simulink library "ddm"  (R2021b)
settings: Solver=VariableStepAuto  StartTime=0.0  StopTime=10.0  RelTol=1e-3
undefined symbols (not defined in the file or in its folder): ENUM_ADASACCSTA_ERROR, ENUM_ADASACCSTA_OFF, ENUM_ADASACCSTA_STANDBY, ENUM_ADASISASTA_OFF, ENUM_ALLOWMOV_ALLOWREADY, ENUM_APS, ENUM_BRKSTA_ERROR, ENUM_BRKSTA_OFF, ENUM_BRKSTA_ON, ENUM_CHGPREACTERRSTA_OBCPRE, ENUM_DCDCFAULTSTA_ANYFAULTLV1, ENUM_DCDCFAULTSTA_ANYFAULTLV2, ENUM_DRIVETRAIN_AWD, ENUM_DRIVETRAIN_FWD, ENUM_DRIVETRAIN_RWD, ENUM_DRSEATSTA_INVALID, ENUM_EDUDRTSTA_NORMAL, ENUM_EPBSTA_APPLIED, ENUM_EPBSTA_RELEASED, ENUM_HVBATTREADYPRE_READY, ENUM_MCUWARN_LV0, ENUM_MCUWARN_LV1, ENUM_MCUWARN_LV2, ENUM_MCUWARN_LV3, ENUM_MCUWARN_NOERROR, ENUM_OBCFAULTSTA_ANYFAULT, ENUM_PAS_R2F2, ENUM_PDFAULT_BATTPDFAIL, ENUM_PDFAULT_DCDCDISABLE, ENUM_PDFAULT_MCUDISABLE, ENUM_PDFAULT_MCUDISCHRG, ENUM_POWERSTA_OFF, ENUM_POWERSTA_ON, ENUM_POWERSTA_READY, ENUM_POWERSTA_STANDBY, ENUM_PRESSINDI_LOW, ENUM_PUFAULT_BATTUPFAIL, ENUM_PUFAULT_DCDCENABLEFAIL, ENUM_PUFAULT_PRECHRGCHKFAIL, ENUM_PUFAULT_SAFETYCHKFAIL, ENUM_PUSTATE_COMPLETED, ENUM_PWRSTASW_OFF, ENUM_PWRSTASW_OFFA, ENUM_PWRSTASW_OFFCHVCHRG, ENUM_PWRSTASW_OFFCLVCHRG, ENUM_PWRSTASW_ON, ENUM_PWRSTASW_ONHVCHRG, ENUM_PWRSTASW_READY, ENUM_PWRSTASW_STANDBY, ENUM_RANGESTA_12IN, ENUM_RANGESTA_12OUT, ENUM_SHIFTCOMMAND_D, ENUM_SHIFTCOMMAND_N, ENUM_SHIFTCOMMAND_P, ENUM_SHIFTCOMMAND_R, ENUM_ZONEMALFUNLV_1ST, ENUM_ZONEMALFUNLV_2ND, ENUM_ZONEMALFUNLV_3RD, ENUM_ZONEMALFUNLV_4TH, ENUM_ZONESPDCTRLMODE_ACC ... (+832)
libraries: hcu_lib x738, $bdroot x26, simulink x7
(part 17 of 25)

== system ddm/DDM/DDM/PMM/SW failure/FR Door switch failure ==
  note: Fail Safe During Detection
  note: Fail Safe After Decision
  note: Release Condition After Decision
  note: Release Condition During Detection
  note: Diagnostics and Fault Handling
  note: Test Detection Criteria
  note: Test Pass Criteria
  task_time_s : Inport
  VPMM_PowerSta_enum : Inport  Port=2
  VPMM_PwrStaSW_enum : Inport  Port=3
  VINP_FRAJARSW : Inport  Port=4
  DTC_clear_request : Inport  Port=5
  Add2 : Sum
  Add3 : Sum
  Add4 : Sum  AccumDataTypeStr=uint16
  Constant{1..2,12..13,31} (5 alike) : Constant  Value=ZERO_INT
  Constant14 : Constant  Value=KDDM_FRDoorSW_s
  Constant28 : Constant  Value=ZERO_FLOAT
  Constant29 : Constant  Value=ONE_INT
  Constant3 : Constant  Value=ONE_INT
  Constant37 : Constant  Value=ENUM_PWRSTASW_OFF
  Constant39 : Constant  Value=KDDM_FRDoorSWPassTO_s
  Constant4 : Constant  Value=KDDM_FRDoorSW_s
  Constant{42,47,52,54} (4 alike) : Constant  Value=TRUE
  Constant45 : Constant  Value=ENUM_POWERSTA_OFF
  Constant49 : Constant  Value=KDDM_FRDoorSW_s
  Constant5 : Constant  Value=KDDM_FRDoorSWDTC_cnt
  Constant50 : Constant  Value=ENUM_PWRSTASW_OFF
  Constant53 : Constant  Value=FALSE
  Constant55 : Constant  Value=FALSE
  Constant56 : Constant  Value=KDDM_FRDoorSWPassSW_flg
  Constant57 : Constant  Value=KDDM_FRDoorSWCFSSW_flg
  Constant58 : Constant  Value=KDDM_FRDoorSWDFSSW_flg
  Constant59 : Constant  Value=KDDM_FRDoorSWDetSW_flg
  Constant6 : Constant  Value=KDDM_FRDoorSWDetTO_s
  Constant60 : Constant  Value=KDDM_FRDoorSWDTC_cnt
  Constant7 : Constant  Value=KDDM_FRDoorSWPassTO_s
  Constant8 : Constant  Value=KDDM_FRDoorSWDetTO_s
  Constant9 : Constant  Value=FALSE
  DTC_Couter1 : hcu_lib/Basic_Blocks/DTC_Couter
  DTC_Info : hcu_lib/Basic_Blocks/DTC_Info
  Data Type Conversion : DataTypeConversion  OutDataTypeStr=uint8
  Data Type Conversion{1..2,7..9} (5 alike) : DataTypeConversion
  Data Type Conversion3 : DataTypeConversion  OutDataTypeStr=uint16
  Data Type Conversion4 : DataTypeConversion  OutDataTypeStr=uint8
  Data Type Conversion5 : DataTypeConversion  OutDataTypeStr=uint32
  Data Type Conversion6 : DataTypeConversion  OutDataTypeStr=uint16
  Divide{,1,7,11,16,20} (6 alike) : Product  Inputs=*/
  Equal10 : RelationalOperator  Operator=~=  OutDataTypeStr=boolean  RndMeth=Simplest
  Equal13 : RelationalOperator  Operator=~=  OutDataTypeStr=boolean  RndMeth=Simplest
  Equal8 : RelationalOperator  Operator===  OutDataTypeStr=boolean  RndMeth=Simplest
  Equal9 : RelationalOperator  Operator=~=  OutDataTypeStr=boolean  RndMeth=Simplest
  Logical Operator1 : Logic  Operator=NOT  AllPortsSameDT=off  OutDataTypeStr=boolean
  Logical Operator{25,28..31} (5 alike) : Logic  AllPortsSameDT=off  OutDataTypeStr=boolean
  Logical Operator27 : Logic  Operator=OR  AllPortsSameDT=off  OutDataTypeStr=boolean
  Logical Operator32 : Logic  Operator=OR  AllPortsSameDT=off  OutDataTypeStr=boolean
  Logical Operator33 : Logic  Operator=OR  AllPortsSameDT=off  OutDataTypeStr=boolean
  Relational Operator : RelationalOperator  Operator=>  OutDataTypeStr=boolean  RndMeth=Simplest
  Relational Operator1 : RelationalOperator  Operator=<=  OutDataTypeStr=boolean  RndMeth=Simplest
  Relational Operator12 : RelationalOperator  OutDataTypeStr=boolean  RndMeth=Simplest
  Relational Operator13 : RelationalOperator  Operator=<  OutDataTypeStr=boolean  RndMeth=Simplest
  Relational Operator2 : RelationalOperator  Operator=>  OutDataTypeStr=boolean  RndMeth=Simplest
  Relational Operator8 : RelationalOperator  Operator=<  OutDataTypeStr=boolean  RndMeth=Simplest
  Relational Operator9 : RelationalOperator  Operator=<=  OutDataTypeStr=boolean  RndMeth=Simplest
  Relay1 : Relay  OnSwitchValue=ONE_INT  OffSwitchValue=ZERO_INT
  SR_Latch2 : hcu_lib/Basic_Blocks/SR_Latch
  SR_Latch5 : hcu_lib/Basic_Blocks/SR_Latch
  Switch{1..3,6,8..9,13} (7 alike) : Switch  Criteria=u2 > Threshold
  Switch{4,7,11..12,15..16} (6 alike) : Switch  Criteria=u2 ~= 0
  Test Detection Criteria1 : hcu_lib/Basic_Blocks/Test Detection Criteria
  Unit Delay{1..3,5..6} (5 alike) : UnitDelay  SampleTime=-1  HasFrameUpgradeWarning=on
  VDDM_FRDoorSWDTC_raw32 : Outport
  VCUFRDoorSta : Outport  Port=2
  wires:
  DTC_clear_request/1 -> [DTC_clear_request]
  VINP_FRAJARSW/1 -> [VINP_FR_AJAR_SW]
  task_time_s/1 -> [task_time_s]
  [VDDM_FRDoorSWCFS_flg] -> Switch11/2
  Constant42/1 -> Switch11/1
  Switch11/1 -> [VCUFRDoorSta]
  Logical Operator27/1 -> Switch15/2
  Constant52/1 -> Switch16/1
  Equal8/1 -> Logical Operator27/1
  [VDDM_FRDoorSWPass_flg] -> Switch16/2
  Constant53/1 -> Switch16/3
  Constant45/1 -> Equal8/2
  Constant55/1 -> Switch15/3
  Switch15/1 -> [VDDM_FRDoorSWCFSRls_flg]
  Switch16/1 -> [VDDM_FRDoorSWDFSRls_flg]
  [DTC_clear_request] -> Logical Operator27/2
  Constant54/1 -> Switch15/1
  [VPMM_PowerSta_enum] -> Equal8/1
  Relay1/1 -> SR_Latch2/1
  [VDDM_FRDoorSWDet_flg] -> Logical Operator31/1
  Logical Operator29/1 -> DTC_Couter1/2
  [VDDM_FRDoorSWCFSRls_flg] -> SR_Latch5/2
  SR_Latch2/1 -> Logical Operator28/2
  SR_Latch5/1 -> Logical Operator30/1
  [VDDM_FRDoorSWDFSRls_flg] -> Logical Operator32/1
  Logical Operator32/1 -> SR_Latch2/2
  DTC_Couter1/2 -> Data Type Conversion4/1
  Logical Operator33/1 -> Logical Operator29/1
  Data Type Conversion4/1 -> [VDDM_FRDoorSWDTC_cnt]  "VDDM_FRDoorSWDTC_cnt"
  [VDDM_FRDoorSWDTC_cnt] -> Relay1/1
  Logical Operator31/1 -> DTC_Couter1/1
  [VDDM_FRDoorSWCFS_flg] -> Logical Operator32/2
  Constant57/1 -> Logical Operator30/2
  DTC_Couter1/1 -> SR_Latch5/1
  Constant59/1 -> Logical Operator31/2
  [VDDM_FRDoorSWCFSRls_flg] -> Logical Operator33/2
  Logical Operator28/1 -> [VDDM_FRDoorSWDFS_flg]
  [VDDM_FRDoorSWPass_flg] -> Logical Operator33/1
  Logical Operator30/1 -> [VDDM_FRDoorSWCFS_flg]
  Constant56/1 -> Logical Operator29/2
  Constant60/1 -> DTC_Couter1/3
  Constant58/1 -> Logical Operator28/1
  [VCUFRDoorSta] -> VCUFRDoorSta/1
  Divide1/1 -> Relational Operator1/2
  Data Type Conversion5/1 -> [VDDM_FRDoorSWHiLoCount_enum]
  Relational Operator1/1 -> [VDDM_FRDoorSWFailcntEN_flg]
  Divide20/1 -> Data Type Conversion9/1
  Add2/1 -> Switch6/3
  [VINP_FR_AJAR_SW] -> Relational Operator/1
  Relational Operator2/1 -> Switch1/2
  Constant31/1 -> Switch6/1
  Unit Delay3/1 -> Equal10/1
  Equal10/1 -> [VDDM_FRDoorSWChange_flg]
  Constant1/1 -> Switch7/3
  Constant29/1 -> Add2/2
  Switch6/1 -> Unit Delay1/1
  Unit Delay1/1 -> Data Type Conversion5/1
  Constant12/1 -> Switch1/1
  Constant37/1 -> Equal13/2
  Switch2/1 -> Data Type Conversion2/1
  Add3/1 -> Data Type Conversion8/1
  Constant4/1 -> Divide/1
  Switch9/1 -> Switch8/1
  Equal13/1 -> Switch7/2
  [VDDM_FRDoorSWfail_cnt] -> Switch1/3
  [VPMM_PwrStaSW_enum] -> Equal13/1
  Switch7/1 -> Unit Delay5/1
  [VDDM_FRDoorSWHiLoCount_enum] -> Relational Operator2/1
  [VDDM_FRDoorSWFailcntEN_flg] -> Switch9/2
  Switch1/1 -> Switch8/3
  Test Detection Criteria1/1 -> [VDDM_FRDoorSWDet_flg]  "VDDM_FRDoorSWDet_flg"
  [VDDM_FRDoorSWHiLoCount_enum] -> Add3/1
  [VDDM_FRDoorSWChange_flg] -> Switch6/2
  [VDDM_FRDoorSWfail_cnt] -> Switch2/1, Relational Operator8/1
  Constant13/1 -> Switch9/3
  Constant14/1 -> Divide1/1
  Relational Operator/1 -> Unit Delay3/1, Equal10/2
  Constant28/1 -> Relational Operator/2
  Constant6/1 -> Divide20/1
  [VDDM_FRDoorSWChange_flg] -> Switch8/2
  Switch8/1 -> Switch7/1
  Divide/1 -> Relational Operator2/2
  Unit Delay5/1 -> Switch4/3, Data Type Conversion7/1
  Unit Delay2/1 -> Relational Operator9/1
  Switch12/1 -> Unit Delay6/1
  Constant3/1 -> Add4/1
  Relational Operator9/1 -> Logical Operator25/2
  Data Type Conversion6/1 -> Relational Operator12/1, [VDDM_FRDoorSWPass_cnt]
  [VDDM_FRDoorSWChange_flg] -> Logical Operator25/1
  Switch3/1 -> Data Type Conversion3/1
  Constant2/1 -> Switch13/3
  [VDDM_FRDoorSWPass_cnt] -> Switch3/1, Relational Operator13/1
  Divide11/1 -> Relational Operator12/2
  Logical Operator1/1 -> Switch13/2
  Logical Operator25/1 -> Logical Operator1/1
  Data Type Conversion/1 -> Switch12/3
  Divide16/1 -> Data Type Conversion1/1
  Constant7/1 -> Divide11/1
  Data Type Conversion3/1 -> Add4/2
  Add4/1 -> Switch13/1
  Equal9/1 -> Switch12/2
  Relational Operator12/1 -> [VDDM_FRDoorSWPass_flg]
  Switch13/1 -> Switch12/1
  Divide7/1 -> Relational Operator9/2
  [VPMM_PwrStaSW_enum] -> Equal9/1
  Constant50/1 -> Equal9/2
  Unit Delay6/1 -> Data Type Conversion6/1
  Constant47/1 -> Data Type Conversion/1
  Constant49/1 -> Divide7/1
  Constant39/1 -> Divide16/1
  [VDDM_FRDoorSWHiLoCount_enum] -> Unit Delay2/1
  VPMM_PowerSta_enum/1 -> [VPMM_PowerSta_enum]
  VPMM_PwrStaSW_enum/1 -> [VPMM_PwrStaSW_enum]
  [VINP_FR_AJAR_SW] -> Switch11/3
  Data Type Conversion9/1 -> Switch2/3, Relational Operator8/2
  Relational Operator8/1 -> Switch2/2
  Data Type Conversion2/1 -> Add3/2
  [VDDM_FRDoorSWHiLoCount_enum] -> Add2/1
  [VDDM_FRDoorSWHiLoCount_enum] -> Relational Operator1/1
  Data Type Conversion7/1 -> [VDDM_FRDoorSWfail_cnt]
  Relational Operator13/1 -> Switch3/2
  Data Type Conversion1/1 -> Switch3/3, Relational Operator13/2
  Data Type Conversion8/1 -> Switch9/1
  DTC_Info/1 -> VDDM_FRDoorSWDTC_raw32/1  "VDDM_FRDoorSWDTC_raw32"
  [VDDM_FRDoorSWPass_flg] -> DTC_Info/2
  [VDDM_FRDoorSWCFS_flg] -> DTC_Info/3
  [VDDM_FRDoorSWDet_flg] -> DTC_Info/1
  [task_time_s] -> Divide1/2
  [task_time_s] -> Divide20/2
  [task_time_s] -> Divide/2
  [task_time_s] -> Divide16/2
  [task_time_s] -> Divide7/2
  [task_time_s] -> Divide11/2
  [task_time_s] -> Test Detection Criteria1/2
  Constant8/1 -> Test Detection Criteria1/4
  Constant5/1 -> Test Detection Criteria1/3
  [DTC_clear_request] -> DTC_Info/4
  [DTC_clear_request] -> Switch4/2
  Switch4/1 -> Test Detection Criteria1/1
  Constant9/1 -> Switch4/1

== system ddm/DDM/DDM/PMM/SW failure/Hood switch failure ==
  note: Test Pass Criteria
  note: Test Detection Criteria
  note: Diagnostics and Fault Handling
  note: Release Condition During Detection
  note: Release Condition After Decision
  note: Fail Safe After Decision
  note: Fail Safe During Detection
  task_time_s : Inport
  VPMM_PowerSta_enum : Inport  Port=2
  VPMM_PwrStaSW_enum : Inport  Port=3
  VINP_HoodSW : Inport  Port=4
  DTC_clear_request : Inport  Port=5
  Add2 : Sum
  Add3 : Sum
  Add4 : Sum  AccumDataTypeStr=uint16
  Constant{1..2,12..13,31} (5 alike) : Constant  Value=ZERO_INT
  Constant14 : Constant  Value=KDDM_HoodSW_s
  Constant28 : Constant  Value=ZERO_FLOAT
  Constant29 : Constant  Value=ONE_INT
  Constant3 : Constant  Value=ONE_INT
  Constant37 : Constant  Value=ENUM_PWRSTASW_OFF
  Constant39 : Constant  Value=KDDM_HoodSWPassTO_s
  Constant4 : Constant  Value=KDDM_HoodSW_s
  Constant{42,47,52,54} (4 alike) : Constant  Value=TRUE
  Constant45 : Constant  Value=ENUM_POWERSTA_OFF
  Constant49 : Constant  Value=KDDM_HoodSW_s
  Constant5 : Constant  Value=KDDM_HoodSWPassTO_s
  Constant50 : Constant  Value=ENUM_PWRSTASW_OFF
  Constant53 : Constant  Value=FALSE
  Constant55 : Constant  Value=FALSE
  Constant56 : Constant  Value=KDDM_HoodSWPassSW_flg
  Constant57 : Constant  Value=KDDM_HoodSWCFSSW_flg
  Constant58 : Constant  Value=KDDM_HoodSWDFSSW_flg
  Constant59 : Constant  Value=KDDM_HoodSWDetSW_flg
  Constant6 : Constant  Value=KDDM_HoodSWDetTO_s
  Constant60 : Constant  Value=KDDM_HoodSWDTC_cnt
  Constant7 : Constant  Value=KDDM_HoodSWDetTO_s
  Constant8 : Constant  Value=KDDM_HoodSWDTC_cnt
  Constant9 : Constant  Value=FALSE
  DTC_Couter1 : hcu_lib/Basic_Blocks/DTC_Couter
  DTC_Info : hcu_lib/Basic_Blocks/DTC_Info
  Data Type Conversion : DataTypeConversion  OutDataTypeStr=uint8
  Data Type Conversion{1..2,7..9} (5 alike) : DataTypeConversion
  Data Type Conversion3 : DataTypeConversion  OutDataTypeStr=uint16
  Data Type Conversion4 : DataTypeConversion  OutDataTypeStr=uint8
  Data Type Conversion5 : DataTypeConversion  OutDataTypeStr=uint32
  Data Type Conversion6 : DataTypeConversion  OutDataTypeStr=uint16
  Divide{,1,7,11,16,20} (6 alike) : Product  Inputs=*/
  Equal10 : RelationalOperator  Operator=~=  OutDataTypeStr=boolean  RndMeth=Simplest
  Equal13 : RelationalOperator  Operator=~=  OutDataTypeStr=boolean  RndMeth=Simplest
  Equal8 : RelationalOperator  Operator===  OutDataTypeStr=boolean  RndMeth=Simplest
  Equal9 : RelationalOperator  Operator=~=  OutDataTypeStr=boolean  RndMeth=Simplest
  Logical Operator1 : Logic  Operator=NOT  AllPortsSameDT=off  OutDataTypeStr=boolean
  Logical Operator{25,28..31} (5 alike) : Logic  AllPortsSameDT=off  OutDataTypeStr=boolean
  Logical Operator27 : Logic  Operator=OR  AllPortsSameDT=off  OutDataTypeStr=boolean
  Logical Operator32 : Logic  Operator=OR  AllPortsSameDT=off  OutDataTypeStr=boolean
  Logical Operator33 : Logic  Operator=OR  AllPortsSameDT=off  OutDataTypeStr=boolean
  Relational Operator : RelationalOperator  Operator=>  OutDataTypeStr=boolean  RndMeth=Simplest
  Relational Operator1 : RelationalOperator  Operator=<=  OutDataTypeStr=boolean  RndMeth=Simplest
  Relational Operator12 : RelationalOperator  OutDataTypeStr=boolean  RndMeth=Simplest
  Relational Operator13 : RelationalOperator  Operator=<  OutDataTypeStr=boolean  RndMeth=Simplest
  Relational Operator2 : RelationalOperator  Operator=>  OutDataTypeStr=boolean  RndMeth=Simplest
  Relational Operator8 : RelationalOperator  Operator=<  OutDataTypeStr=boolean  RndMeth=Simplest
  Relational Operator9 : RelationalOperator  Operator=<=  OutDataTypeStr=boolean  RndMeth=Simplest
  Relay1 : Relay  OnSwitchValue=ONE_INT  OffSwitchValue=ZERO_INT
  SR_Latch2 : hcu_lib/Basic_Blocks/SR_Latch
  SR_Latch5 : hcu_lib/Basic_Blocks/SR_Latch
  Switch{1..3,6,8..9,13} (7 alike) : Switch  Criteria=u2 > Threshold
  Switch{4,7,11..12,15..16} (6 alike) : Switch  Criteria=u2 ~= 0
  Test Detection Criteria1 : hcu_lib/Basic_Blocks/Test Detection Criteria
  Unit Delay{1..3,5..6} (5 alike) : UnitDelay  SampleTime=-1  HasFrameUpgradeWarning=on
  VDDM_HoodSWDTC_raw32 : Outport
  VCUHoodSWSta : Outport  Port=2
  wires:
  [VDDM_HoodSWHiLoCount_enum] -> Unit Delay2/1
  Constant39/1 -> Divide16/1
  Constant49/1 -> Divide7/1
  Constant47/1 -> Data Type Conversion/1
  Unit Delay6/1 -> Data Type Conversion6/1
  Constant50/1 -> Equal9/2
  [VPMM_PwrStaSW_enum] -> Equal9/1
  Divide7/1 -> Relational Operator9/2
  Switch13/1 -> Switch12/1
  Relational Operator12/1 -> [VDDM_HoodSWPass_flg]
  Equal9/1 -> Switch12/2
  Add4/1 -> Switch13/1
  Data Type Conversion3/1 -> Add4/2
  Constant5/1 -> Divide11/1
  Divide16/1 -> Data Type Conversion1/1
  Data Type Conversion/1 -> Switch12/3
  Logical Operator25/1 -> Logical Operator1/1
  Logical Operator1/1 -> Switch13/2
  Divide11/1 -> Relational Operator12/2
  [VDDM_HoodSWPass_cnt] -> Relational Operator13/1, Switch3/1
  Constant2/1 -> Switch13/3
  Switch3/1 -> Data Type Conversion3/1
  [VDDM_HoodSWChange_flg] -> Logical Operator25/1
  Data Type Conversion6/1 -> [VDDM_HoodSWPass_cnt], Relational Operator12/1
  Relational Operator9/1 -> Logical Operator25/2
  Constant3/1 -> Add4/1
  Switch12/1 -> Unit Delay6/1
  Unit Delay2/1 -> Relational Operator9/1
  Unit Delay5/1 -> Data Type Conversion7/1, Switch4/3
  Divide/1 -> Relational Operator2/2
  Switch8/1 -> Switch7/1
  [VDDM_HoodSWChange_flg] -> Switch8/2
  Constant6/1 -> Divide20/1
  Constant28/1 -> Relational Operator/2
  Relational Operator/1 -> Equal10/2, Unit Delay3/1
  Constant14/1 -> Divide1/1
  Constant13/1 -> Switch9/3
  [VDDM_HoodSWfail_cnt] -> Relational Operator8/1, Switch2/1
  [VDDM_HoodSWChange_flg] -> Switch6/2
  [VDDM_HoodSWHiLoCount_enum] -> Add3/1
  Test Detection Criteria1/1 -> [VDDM_HoodSWDet_flg]  "VDDM_HoodSWDet_flg"
  Switch1/1 -> Switch8/3
  [VDDM_HoodSWFailcntEN_flg] -> Switch9/2
  [VDDM_HoodSWHiLoCount_enum] -> Relational Operator2/1
  Switch7/1 -> Unit Delay5/1
  [VPMM_PwrStaSW_enum] -> Equal13/1
  [VDDM_HoodSWfail_cnt] -> Switch1/3
  Equal13/1 -> Switch7/2
  Switch9/1 -> Switch8/1
  Constant4/1 -> Divide/1
  Add3/1 -> Data Type Conversion8/1
  Switch2/1 -> Data Type Conversion2/1
  Constant37/1 -> Equal13/2
  Constant12/1 -> Switch1/1
  Unit Delay1/1 -> Data Type Conversion5/1
  Switch6/1 -> Unit Delay1/1
  Constant29/1 -> Add2/2
  Constant1/1 -> Switch7/3
  Equal10/1 -> [VDDM_HoodSWChange_flg]
  Unit Delay3/1 -> Equal10/1
  Constant31/1 -> Switch6/1
  Relational Operator2/1 -> Switch1/2
  [VINP_HoodSWGPIO_flg] -> Relational Operator/1
  Add2/1 -> Switch6/3
  Divide20/1 -> Data Type Conversion9/1
  Relational Operator1/1 -> [VDDM_HoodSWFailcntEN_flg]
  Data Type Conversion5/1 -> [VDDM_HoodSWHiLoCount_enum]
  Divide1/1 -> Relational Operator1/2
  [VCUHoodSWSta] -> VCUHoodSWSta/1
  Constant58/1 -> Logical Operator28/1
  Constant60/1 -> DTC_Couter1/3
  Constant56/1 -> Logical Operator29/2
  Logical Operator30/1 -> [VDDM_HoodSWCFS_flg]
  [VDDM_HoodSWPass_flg] -> Logical Operator33/1
  Logical Operator28/1 -> [VDDM_HoodSWDFS_flg]
  [VDDM_HoodSWCFSRls_flg] -> Logical Operator33/2
  Constant59/1 -> Logical Operator31/2
  DTC_Couter1/1 -> SR_Latch5/1
  Constant57/1 -> Logical Operator30/2
  [VDDM_HoodSWCFS_flg] -> Logical Operator32/2
  Logical Operator31/1 -> DTC_Couter1/1
  [VDDM_HoodSWDTC_cnt] -> Relay1/1
  Data Type Conversion4/1 -> [VDDM_HoodSWDTC_cnt]  "VDDM_HoodSWDTC_cnt"
  Logical Operator33/1 -> Logical Operator29/1
  DTC_Couter1/2 -> Data Type Conversion4/1
  Logical Operator32/1 -> SR_Latch2/2
  [VDDM_HoodSWDFSRls_flg] -> Logical Operator32/1
  SR_Latch5/1 -> Logical Operator30/1
  SR_Latch2/1 -> Logical Operator28/2
  [VDDM_HoodSWCFSRls_flg] -> SR_Latch5/2
  Logical Operator29/1 -> DTC_Couter1/2
  [VDDM_HoodSWDet_flg] -> Logical Operator31/1
  Relay1/1 -> SR_Latch2/1
  [VPMM_PowerSta_enum] -> Equal8/1
  Constant54/1 -> Switch15/1
  [DTC_clear_request] -> Logical Operator27/2
  Switch16/1 -> [VDDM_HoodSWDFSRls_flg]
  Switch15/1 -> [VDDM_HoodSWCFSRls_flg]
  Constant55/1 -> Switch15/3
  Constant45/1 -> Equal8/2
  Constant53/1 -> Switch16/3
  [VDDM_HoodSWPass_flg] -> Switch16/2
  Equal8/1 -> Logical Operator27/1
  Constant52/1 -> Switch16/1
  Logical Operator27/1 -> Switch15/2
  Switch11/1 -> [VCUHoodSWSta]
  Constant42/1 -> Switch11/1
  [VDDM_HoodSWCFS_flg] -> Switch11/2
  task_time_s/1 -> [task_time_s]
  VINP_HoodSW/1 -> [VINP_HoodSWGPIO_flg]
  DTC_clear_request/1 -> [DTC_clear_request]
  VPMM_PowerSta_enum/1 -> [VPMM_PowerSta_enum]
  VPMM_PwrStaSW_enum/1 -> [VPMM_PwrStaSW_enum]
  [VINP_HoodSWGPIO_flg] -> Switch11/3
  Data Type Conversion9/1 -> Relational Operator8/2, Switch2/3
  Relational Operator8/1 -> Switch2/2
  Data Type Conversion2/1 -> Add3/2
  [VDDM_HoodSWHiLoCount_enum] -> Relational Operator1/1
  [VDDM_HoodSWHiLoCount_enum] -> Add2/1
  Data Type Conversion7/1 -> [VDDM_HoodSWfail_cnt]
  Relational Operator13/1 -> Switch3/2
  Data Type Conversion1/1 -> Relational Operator13/2, Switch3/3
  Data Type Conversion8/1 -> Switch9/1
  DTC_Info/1 -> VDDM_HoodSWDTC_raw32/1  "VDDM_HoodSWDTC_raw32"
  [VDDM_HoodSWPass_flg] -> DTC_Info/2
  [VDDM_HoodSWCFS_flg] -> DTC_Info/3
  [VDDM_HoodSWDet_flg] -> DTC_Info/1
  [task_time_s] -> Divide20/2
  [task_time_s] -> Divide1/2
  [task_time_s] -> Divide/2
  [task_time_s] -> Divide16/2
  [task_time_s] -> Divide7/2
  [task_time_s] -> Divide11/2
  [task_time_s] -> Test Detection Criteria1/2
  Constant7/1 -> Test Detection Criteria1/4
  Constant8/1 -> Test Detection Criteria1/3
  [DTC_clear_request] -> DTC_Info/4
  [DTC_clear_request] -> Switch4/2
  Switch4/1 -> Test Detection Criteria1/1
  Constant9/1 -> Switch4/1

== system ddm/DDM/DDM/PMM/SW failure/RL Door switch failure ==
  note: Fail Safe During Detection
  note: Fail Safe After Decision
  note: Release Condition After Decision
  note: Release Condition During Detection
  note: Diagnostics and Fault Handling
  note: Test Detection Criteria
  note: Test Pass Criteria
  task_time_s : Inport
  VPMM_PowerSta_enum : Inport  Port=2
  VPMM_PwrStaSW_enum : Inport  Port=3
  VINP_RLAJARSW : Inport  Port=4
  DTC_clear_request : Inport  Port=5
  Add2 : Sum
  Add3 : Sum
  Add4 : Sum  AccumDataTypeStr=uint16
  Constant{1..2,12..13,31} (5 alike) : Constant  Value=ZERO_INT
  Constant14 : Constant  Value=KDDM_RLDoorSW_s
  Constant28 : Constant  Value=ZERO_FLOAT
  Constant29 : Constant  Value=ONE_INT
  Constant3 : Constant  Value=ONE_INT
  Constant37 : Constant  Value=ENUM_PWRSTASW_OFF
  Constant39 : Constant  Value=KDDM_RLDoorSWPassTO_s
  Constant4 : Constant  Value=KDDM_RLDoorSW_s
  Constant{42,47,52,54} (4 alike) : Constant  Value=TRUE
  Constant45 : Constant  Value=ENUM_POWERSTA_OFF
  Constant49 : Constant  Value=KDDM_RLDoorSW_s
  Constant5 : Constant  Value=KDDM_RLDoorSWDTC_cnt
  Constant50 : Constant  Value=ENUM_PWRSTASW_OFF
  Constant53 : Constant  Value=FALSE
  Constant55 : Constant  Value=FALSE
  Constant56 : Constant  Value=KDDM_RLDoorSWPassSW_flg
  Constant57 : Constant  Value=KDDM_RLDoorSWCFSSW_flg
  Constant58 : Constant  Value=KDDM_RLDoorSWDFSSW_flg
  Constant59 : Constant  Value=KDDM_RLDoorSWDetSW_flg
  Constant6 : Constant  Value=KDDM_RLDoorSWDetTO_s
  Constant60 : Constant  Value=KDDM_RLDoorSWDTC_cnt
  Constant7 : Constant  Value=KDDM_RLDoorSWPassTO_s
  Constant8 : Constant  Value=KDDM_RLDoorSWDetTO_s
  Constant9 : Constant  Value=FALSE
  DTC_Couter1 : hcu_lib/Basic_Blocks/DTC_Couter
  DTC_Info : hcu_lib/Basic_Blocks/DTC_Info
  Data Type Conversion : DataTypeConversion  OutDataTypeStr=uint8
  Data Type Conversion{1..2,7..10} (6 alike) : DataTypeConversion
  Data Type Conversion3 : DataTypeConversion  OutDataTypeStr=uint16
  Data Type Conversion4 : DataTypeConversion  OutDataTypeStr=uint8
  Data Type Conversion5 : DataTypeConversion  OutDataTypeStr=uint32
  Data Type Conversion6 : DataTypeConversion  OutDataTypeStr=uint16
  Divide{,1,7,11,16,20} (6 alike) : Product  Inputs=*/
  Equal10 : RelationalOperator  Operator=~=  OutDataTypeStr=boolean  RndMeth=Simplest
  Equal13 : RelationalOperator  Operator=~=  OutDataTypeStr=boolean  RndMeth=Simplest
  Equal8 : RelationalOperator  Operator===  OutDataTypeStr=boolean  RndMeth=Simplest
  Equal9 : RelationalOperator  Operator=~=  OutDataTypeStr=boolean  RndMeth=Simplest
  Logical Operator1 : Logic  Operator=NOT  AllPortsSameDT=off  OutDataTypeStr=boolean
  Logical Operator{25,28..31} (5 alike) : Logic  AllPortsSameDT=off  OutDataTypeStr=boolean
  Logical Operator27 : Logic  Operator=OR  AllPortsSameDT=off  OutDataTypeStr=boolean
  Logical Operator32 : Logic  Operator=OR  AllPortsSameDT=off  OutDataTypeStr=boolean
  Logical Operator33 : Logic  Operator=OR  AllPortsSameDT=off  OutDataTypeStr=boolean
  Relational Operator : RelationalOperator  Operator=>  OutDataTypeStr=boolean  RndMeth=Simplest
  Relational Operator1 : RelationalOperator  Operator=<=  OutDataTypeStr=boolean  RndMeth=Simplest
  Relational Operator12 : RelationalOperator  OutDataTypeStr=boolean  RndMeth=Simplest
  Relational Operator13 : RelationalOperator  Operator=<  OutDataTypeStr=boolean  RndMeth=Simplest
  Relational Operator2 : RelationalOperator  Operator=>  OutDataTypeStr=boolean  RndMeth=Simplest
  Relational Operator8 : RelationalOperator  Operator=<  OutDataTypeStr=boolean  RndMeth=Simplest
  Relational Operator9 : RelationalOperator  Operator=<=  OutDataTypeStr=boolean  RndMeth=Simplest
  Relay1 : Relay  OnSwitchValue=ONE_INT  OffSwitchValue=ZERO_INT
  SR_Latch2 : hcu_lib/Basic_Blocks/SR_Latch
  SR_Latch5 : hcu_lib/Basic_Blocks/SR_Latch
  Switch{1..3,6,8..9,13} (7 alike) : Switch  Criteria=u2 > Threshold
  Switch{4,7,11..12,15..16} (6 alike) : Switch  Criteria=u2 ~= 0
  Test Detection Criteria1 : hcu_lib/Basic_Blocks/Test Detection Criteria
  Unit Delay{1..3,5..6} (5 alike) : UnitDelay  SampleTime=-1  HasFrameUpgradeWarning=on
  VDDM_RLDoorSWDTC_raw32 : Outport
  VCURLDoorSta : Outport  Port=2
  wires:
  DTC_clear_request/1 -> [DTC_clear_request]
  VINP_RLAJARSW/1 -> [VINP_RL_AJAR_SW]
  task_time_s/1 -> [task_time_s]
  [VDDM_RLDoorSWCFS_flg] -> Switch11/2
  Constant42/1 -> Switch11/1
  Switch11/1 -> [VCURLDoorSta]
  Logical Operator27/1 -> Switch15/2
  Constant52/1 -> Switch16/1
  Equal8/1 -> Logical Operator27/1
  [VDDM_RLDoorSWPass_flg] -> Switch16/2
  Constant53/1 -> Switch16/3
  Constant45/1 -> Equal8/2
  Constant55/1 -> Switch15/3
  Switch15/1 -> [VDDM_RLDoorSWCFSRls_flg]
  Switch16/1 -> [VDDM_RLDoorSWDFSRls_flg]
  [DTC_clear_request] -> Logical Operator27/2
  Constant54/1 -> Switch15/1
  [VPMM_PowerSta_enum] -> Equal8/1
  Relay1/1 -> SR_Latch2/1
  [VDDM_RLDoorSWDet_flg] -> Logical Operator31/1
  Logical Operator29/1 -> DTC_Couter1/2
  [VDDM_RLDoorSWCFSRls_flg] -> SR_Latch5/2
  SR_Latch2/1 -> Logical Operator28/2
  SR_Latch5/1 -> Logical Operator30/1
  [VDDM_RLDoorSWDFSRls_flg] -> Logical Operator32/1
  Logical Operator32/1 -> SR_Latch2/2
  DTC_Couter1/2 -> Data Type Conversion4/1
  Logical Operator33/1 -> Logical Operator29/1
  Data Type Conversion4/1 -> [VDDM_RLDoorSWDTC_cnt]
  [VDDM_RLDoorSWDTC_cnt] -> Relay1/1
  Logical Operator31/1 -> DTC_Couter1/1
  [VDDM_RLDoorSWCFS_flg] -> Logical Operator32/2
  Constant57/1 -> Logical Operator30/2
  DTC_Couter1/1 -> SR_Latch5/1
  Constant59/1 -> Logical Operator31/2
  [VDDM_RLDoorSWCFSRls_flg] -> Logical Operator33/2
  Logical Operator28/1 -> [VDDM_RLDoorSWDFS_flg]
  [VDDM_RLDoorSWPass_flg] -> Logical Operator33/1
  Logical Operator30/1 -> [VDDM_RLDoorSWCFS_flg]  "VDDM_RLDoorSWCFS_flg"
  Constant56/1 -> Logical Operator29/2
  Constant60/1 -> DTC_Couter1/3
  Constant58/1 -> Logical Operator28/1
  [VCURLDoorSta] -> VCURLDoorSta/1
  Divide1/1 -> Relational Operator1/2
  Data Type Conversion5/1 -> [VDDM_RLDoorSWHiLoCount_enum]
  Relational Operator1/1 -> [VDDM_RLDoorSWFailcntEN_flg]
  Divide20/1 -> Data Type Conversion9/1
  Add2/1 -> Switch6/3
  [VINP_RL_AJAR_SW] -> Relational Operator/1
  Relational Operator2/1 -> Switch1/2
  Constant31/1 -> Switch6/1
  Unit Delay3/1 -> Equal10/1
  Equal10/1 -> [VDDM_RLDoorSWChange_flg]
  Constant1/1 -> Switch7/3
  Constant29/1 -> Add2/2
  Switch6/1 -> Unit Delay1/1
  Unit Delay1/1 -> Data Type Conversion5/1
  Constant12/1 -> Switch1/1
  Constant37/1 -> Equal13/2
  Switch2/1 -> Data Type Conversion2/1
  Constant4/1 -> Divide/1
  Switch9/1 -> Switch8/1
  Equal13/1 -> Switch7/2
  [VDDM_RLDoorSWfail_cnt] -> Switch1/3
  [VPMM_PwrStaSW_enum] -> Equal13/1
  Switch7/1 -> Unit Delay5/1
  [VDDM_RLDoorSWHiLoCount_enum] -> Relational Operator2/1
  [VDDM_RLDoorSWFailcntEN_flg] -> Switch9/2
  Switch1/1 -> Switch8/3
  Test Detection Criteria1/1 -> [VDDM_RLDoorSWDet_flg]  "VDDM_RLDoorSWDet_flg"
  Constant8/1 -> Test Detection Criteria1/4
  [VDDM_RLDoorSWHiLoCount_enum] -> Add3/1
  [VDDM_RLDoorSWChange_flg] -> Switch6/2
  [VDDM_RLDoorSWfail_cnt] -> Switch2/1, Relational Operator8/1
  Constant13/1 -> Switch9/3
  Constant14/1 -> Divide1/1
  Relational Operator/1 -> Unit Delay3/1, Equal10/2
  Constant28/1 -> Relational Operator/2
  Constant6/1 -> Divide20/1
  [VDDM_RLDoorSWChange_flg] -> Switch8/2
  Switch8/1 -> Switch7/1
  Divide/1 -> Relational Operator2/2
  Unit Delay5/1 -> Data Type Conversion10/1
  Unit Delay2/1 -> Relational Operator9/1
  Switch12/1 -> Unit Delay6/1
  Constant3/1 -> Add4/1
  Relational Operator9/1 -> Logical Operator25/2
  Data Type Conversion6/1 -> Relational Operator12/1, [VDDM_RLDoorSWPass_cnt]
  [VDDM_RLDoorSWChange_flg] -> Logical Operator25/1
  Switch3/1 -> Data Type Conversion3/1
  Constant2/1 -> Switch13/3
  [VDDM_RLDoorSWPass_cnt] -> Switch3/1, Relational Operator13/1
  Divide11/1 -> Relational Operator12/2
  Logical Operator1/1 -> Switch13/2
  Logical Operator25/1 -> Logical Operator1/1
  Data Type Conversion1/1 -> Switch3/2
  Data Type Conversion/1 -> Switch12/3
  Divide16/1 -> Data Type Conversion7/1
  Constant7/1 -> Divide11/1
  Data Type Conversion3/1 -> Add4/2
  Add4/1 -> Switch13/1
  Equal9/1 -> Switch12/2
  Relational Operator12/1 -> [VDDM_RLDoorSWPass_flg]
  Relational Operator13/1 -> Data Type Conversion1/1
  Switch13/1 -> Switch12/1
  Divide7/1 -> Relational Operator9/2
  [VPMM_PwrStaSW_enum] -> Equal9/1
  Constant50/1 -> Equal9/2
  Unit Delay6/1 -> Data Type Conversion6/1
  Constant47/1 -> Data Type Conversion/1
  Constant49/1 -> Divide7/1
  Constant39/1 -> Divide16/1
  [VDDM_RLDoorSWHiLoCount_enum] -> Unit Delay2/1
  VPMM_PwrStaSW_enum/1 -> [VPMM_PwrStaSW_enum]
  VPMM_PowerSta_enum/1 -> [VPMM_PowerSta_enum]
  [VINP_RL_AJAR_SW] -> Switch11/3
  Data Type Conversion9/1 -> Switch2/3, Relational Operator8/2
  Relational Operator8/1 -> Switch2/2
  Data Type Conversion2/1 -> Add3/2
  [VDDM_RLDoorSWHiLoCount_enum] -> Relational Operator1/1
  [VDDM_RLDoorSWHiLoCount_enum] -> Add2/1
  Data Type Conversion7/1 -> Switch3/3, Relational Operator13/2
  Add3/1 -> Data Type Conversion8/1
  Data Type Conversion8/1 -> Switch9/1
  [VDDM_RLDoorSWPass_flg] -> DTC_Info/2
  [VDDM_RLDoorSWCFS_flg] -> DTC_Info/3
  DTC_Info/1 -> VDDM_RLDoorSWDTC_raw32/1  "VDDM_RLDoorSWDTC_raw32"
  [VDDM_RLDoorSWDet_flg] -> DTC_Info/1
  [task_time_s] -> Divide1/2
  [task_time_s] -> Divide20/2
  [task_time_s] -> Divide/2
  [task_time_s] -> Test Detection Criteria1/2
  [task_time_s] -> Divide16/2
  [task_time_s] -> Divide7/2
  [task_time_s] -> Divide11/2
  Constant5/1 -> Test Detection Criteria1/3
  [DTC_clear_request] -> DTC_Info/4
  [DTC_clear_request] -> Switch4/2
  Switch4/1 -> Test Detection Criteria1/1
  Data Type Conversion10/1 -> [VDDM_RLDoorSWfail_cnt], Switch4/3
  Constant9/1 -> Switch4/1

== system ddm/DDM/DDM/PMM/SW failure/RR Door switch failure ==
  note: Test Pass Criteria
  note: Test Detection Criteria
  note: Diagnostics and Fault Handling
  note: Release Condition During Detection
  note: Release Condition After Decision
  note: Fail Safe After Decision
  note: Fail Safe During Detection
  task_time_s : Inport
  VPMM_PowerSta_enum : Inport  Port=2
  VPMM_PwrStaSW_enum : Inport  Port=3
  VINP_RRAJARSW : Inport  Port=4
  DTC_clear_request : Inport  Port=5
  Add2 : Sum
  Add3 : Sum
  Add4 : Sum  AccumDataTypeStr=uint16
  Constant{1..2,12..13,31} (5 alike) : Constant  Value=ZERO_INT
  Constant14 : Constant  Value=KDDM_RRDoorSW_s
  Constant28 : Constant  Value=ZERO_FLOAT
  Constant29 : Constant  Value=ONE_INT
  Constant3 : Constant  Value=ONE_INT
  Constant37 : Constant  Value=ENUM_PWRSTASW_OFF
  Constant39 : Constant  Value=KDDM_RRDoorSWPassTO_s
  Constant4 : Constant  Value=KDDM_RRDoorSW_s
  Constant{42,47,52,54} (4 alike) : Constant  Value=TRUE
  Constant45 : Constant  Value=ENUM_POWERSTA_OFF
  Constant49 : Constant  Value=KDDM_RRDoorSW_s
  Constant5 : Constant  Value=KDDM_RRDoorSWDTC_cnt
  Constant50 : Constant  Value=ENUM_PWRSTASW_OFF
  Constant53 : Constant  Value=FALSE
  Constant55 : Constant  Value=FALSE
  Constant56 : Constant  Value=KDDM_RRDoorSWPassSW_flg
  Constant57 : Constant  Value=KDDM_RRDoorSWCFSSW_flg
  Constant58 : Constant  Value=KDDM_RRDoorSWDFSSW_flg
  Constant59 : Constant  Value=KDDM_RRDoorSWDetSW_flg
  Constant6 : Constant  Value=KDDM_RRDoorSWDetTO_s
  Constant60 : Constant  Value=KDDM_RRDoorSWDTC_cnt
  Constant7 : Constant  Value=KDDM_RRDoorSWPassTO_s
  Constant8 : Constant  Value=KDDM_RRDoorSWDetTO_s
  Constant9 : Constant  Value=FALSE
  DTC_Couter1 : hcu_lib/Basic_Blocks/DTC_Couter
  DTC_Info : hcu_lib/Basic_Blocks/DTC_Info
  Data Type Conversion : DataTypeConversion  OutDataTypeStr=uint8
  Data Type Conversion{1..2,7..9} (5 alike) : DataTypeConversion
  Data Type Conversion3 : DataTypeConversion  OutDataTypeStr=uint16
  Data Type Conversion4 : DataTypeConversion  OutDataTypeStr=uint8
  Data Type Conversion5 : DataTypeConversion  OutDataTypeStr=uint32
  Data Type Conversion6 : DataTypeConversion  OutDataTypeStr=uint16
  Divide{,1,7,11,16,20} (6 alike) : Product  Inputs=*/
  Equal10 : RelationalOperator  Operator=~=  OutDataTypeStr=boolean  RndMeth=Simplest
  Equal13 : RelationalOperator  Operator=~=  OutDataTypeStr=boolean  RndMeth=Simplest
  Equal8 : RelationalOperator  Operator===  OutDataTypeStr=boolean  RndMeth=Simplest
  Equal9 : RelationalOperator  Operator=~=  OutDataTypeStr=boolean  RndMeth=Simplest
  Logical Operator1 : Logic  Operator=NOT  AllPortsSameDT=off  OutDataTypeStr=boolean
  Logical Operator{25,28..31} (5 alike) : Logic  AllPortsSameDT=off  OutDataTypeStr=boolean
  Logical Operator27 : Logic  Operator=OR  AllPortsSameDT=off  OutDataTypeStr=boolean
  Logical Operator32 : Logic  Operator=OR  AllPortsSameDT=off  OutDataTypeStr=boolean
  Logical Operator33 : Logic  Operator=OR  AllPortsSameDT=off  OutDataTypeStr=boolean
  Relational Operator : RelationalOperator  Operator=>  OutDataTypeStr=boolean  RndMeth=Simplest
  Relational Operator1 : RelationalOperator  Operator=<=  OutDataTypeStr=boolean  RndMeth=Simplest
  Relational Operator12 : RelationalOperator  OutDataTypeStr=boolean  RndMeth=Simplest
  Relational Operator13 : RelationalOperator  Operator=<  OutDataTypeStr=boolean  RndMeth=Simplest
  Relational Operator2 : RelationalOperator  Operator=>  OutDataTypeStr=boolean  RndMeth=Simplest
  Relational Operator8 : RelationalOperator  Operator=<  OutDataTypeStr=boolean  RndMeth=Simplest
  Relational Operator9 : RelationalOperator  Operator=<=  OutDataTypeStr=boolean  RndMeth=Simplest
  Relay1 : Relay  OnSwitchValue=ONE_INT  OffSwitchValue=ZERO_INT
  SR_Latch2 : hcu_lib/Basic_Blocks/SR_Latch
  SR_Latch5 : hcu_lib/Basic_Blocks/SR_Latch
  Switch{1..3,6,8..9,13} (7 alike) : Switch  Criteria=u2 > Threshold
  Switch{4,7,11..12,15..16} (6 alike) : Switch  Criteria=u2 ~= 0
  Test Detection Criteria1 : hcu_lib/Basic_Blocks/Test Detection Criteria
  Unit Delay{1..3,5..6} (5 alike) : UnitDelay  SampleTime=-1  HasFrameUpgradeWarning=on
  VDDM_RRDoorSWDTC_raw32 : Outport
  VCURRDoorSta : Outport  Port=2
  wires:
  [VDDM_RRDoorSWHiLoCount_enum] -> Unit Delay2/1
  Constant39/1 -> Divide16/1
  Constant49/1 -> Divide7/1
  Constant47/1 -> Data Type Conversion/1
  Unit Delay6/1 -> Data Type Conversion6/1
  Constant50/1 -> Equal9/2
  [VPMM_PwrStaSW_enum] -> Equal9/1
  Divide7/1 -> Relational Operator9/2
  Switch13/1 -> Switch12/1
  Relational Operator12/1 -> [VDDM_RRDoorSWPass_flg]
  Equal9/1 -> Switch12/2
  Add4/1 -> Switch13/1
  Data Type Conversion3/1 -> Add4/2
  Constant7/1 -> Divide11/1
  Divide16/1 -> Data Type Conversion1/1
  Data Type Conversion/1 -> Switch12/3
  Logical Operator25/1 -> Logical Operator1/1
  Logical Operator1/1 -> Switch13/2
  Divide11/1 -> Relational Operator12/2
  [VDDM_RRDoorSWPass_cnt] -> Relational Operator13/1, Switch3/1
  Constant2/1 -> Switch13/3
  Switch3/1 -> Data Type Conversion3/1
  [VDDM_RRDoorSWChange_flg] -> Logical Operator25/1
  Data Type Conversion6/1 -> [VDDM_RRDoorSWPass_cnt], Relational Operator12/1
  Relational Operator9/1 -> Logical Operator25/2
  Constant3/1 -> Add4/1
  Switch12/1 -> Unit Delay6/1
  Unit Delay2/1 -> Relational Operator9/1
  Unit Delay5/1 -> Switch4/3, Data Type Conversion7/1
  Divide/1 -> Relational Operator2/2
  Switch8/1 -> Switch7/1
  [VDDM_RRDoorSWChange_flg] -> Switch8/2
  Constant6/1 -> Divide20/1
  Constant28/1 -> Relational Operator/2
  Relational Operator/1 -> Equal10/2, Unit Delay3/1
  Constant14/1 -> Divide1/1
  Constant13/1 -> Switch9/3
  [VDDM_RRDoorSWfail_cnt] -> Relational Operator8/1, Switch2/1
  [VDDM_RRDoorSWChange_flg] -> Switch6/2
  [VDDM_RRDoorSWHiLoCount_enum] -> Add3/1
  Constant8/1 -> Test Detection Criteria1/4
  Test Detection Criteria1/1 -> [VDDM_RRDoorSWDet_flg]  "VDDM_RRDoorSWDet_flg"
  Switch1/1 -> Switch8/3
  [VDDM_RRDoorSWFailcntEN_flg] -> Switch9/2
  [VDDM_RRDoorSWHiLoCount_enum] -> Relational Operator2/1
  Switch7/1 -> Unit Delay5/1
  [VPMM_PwrStaSW_enum] -> Equal13/1
  [VDDM_RRDoorSWfail_cnt] -> Switch1/3
  Equal13/1 -> Switch7/2
  Switch9/1 -> Switch8/1
  Constant4/1 -> Divide/1
  Add3/1 -> Data Type Conversion8/1
  Switch2/1 -> Data Type Conversion2/1
  Constant37/1 -> Equal13/2
  Constant12/1 -> Switch1/1
  Unit Delay1/1 -> Data Type Conversion5/1
  Switch6/1 -> Unit Delay1/1
  Constant29/1 -> Add2/2
  Constant1/1 -> Switch7/3
  Equal10/1 -> [VDDM_RRDoorSWChange_flg]
  Unit Delay3/1 -> Equal10/1
  Constant31/1 -> Switch6/1
  Relational Operator2/1 -> Switch1/2
  [VINP_RR_AJAR_SW] -> Relational Operator/1
  Add2/1 -> Switch6/3
  Divide20/1 -> Data Type Conversion9/1
  Relational Operator1/1 -> [VDDM_RRDoorSWFailcntEN_flg]
  Data Type Conversion5/1 -> [VDDM_RRDoorSWHiLoCount_enum]
  Divide1/1 -> Relational Operator1/2
  [VCURRDoorSta] -> VCURRDoorSta/1
  Constant58/1 -> Logical Operator28/1
  Constant60/1 -> DTC_Couter1/3
  Constant56/1 -> Logical Operator29/2
  Logical Operator30/1 -> [VDDM_RRDoorSWCFS_flg]
  [VDDM_RRDoorSWPass_flg] -> Logical Operator33/1
  Logical Operator28/1 -> [VDDM_RRDoorSWDFS_flg]
  [VDDM_RRDoorSWCFSRls_flg] -> Logical Operator33/2
  Constant59/1 -> Logical Operator31/2
  DTC_Couter1/1 -> SR_Latch5/1
  Constant57/1 -> Logical Operator30/2
  [VDDM_RRDoorSWCFS_flg] -> Logical Operator32/2
  Logical Operator31/1 -> DTC_Couter1/1
  [VDDM_RRDoorSWDTC_cnt] -> Relay1/1
  Data Type Conversion4/1 -> [VDDM_RRDoorSWDTC_cnt]  "VDDM_RRDoorSWDTC_cnt"
  Logical Operator33/1 -> Logical Operator29/1
  DTC_Couter1/2 -> Data Type Conversion4/1
  Logical Operator32/1 -> SR_Latch2/2
  [VDDM_RRDoorSWDFSRls_flg] -> Logical Operator32/1
  SR_Latch5/1 -> Logical Operator30/1
  SR_Latch2/1 -> Logical Operator28/2
  [VDDM_RRDoorSWCFSRls_flg] -> SR_Latch5/2
  Logical Operator29/1 -> DTC_Couter1/2
  [VDDM_RRDoorSWDet_flg] -> Logical Operator31/1
  Relay1/1 -> SR_Latch2/1
  [VPMM_PowerSta_enum] -> Equal8/1
  Constant54/1 -> Switch15/1
  [DTC_clear_request] -> Logical Operator27/2
  Switch16/1 -> [VDDM_RRDoorSWDFSRls_flg]
  Switch15/1 -> [VDDM_RRDoorSWCFSRls_flg]
  Constant55/1 -> Switch15/3
  Constant45/1 -> Equal8/2
  Constant53/1 -> Switch16/3
  [VDDM_RRDoorSWPass_flg] -> Switch16/2
  Equal8/1 -> Logical Operator27/1
  Constant52/1 -> Switch16/1
  Logical Operator27/1 -> Switch15/2
  Switch11/1 -> [VCURRDoorSta]
  Constant42/1 -> Switch11/1
  [VDDM_RRDoorSWCFS_flg] -> Switch11/2
  task_time_s/1 -> [task_time_s]
  VINP_RRAJARSW/1 -> [VINP_RR_AJAR_SW]
  DTC_clear_request/1 -> [DTC_clear_request]
  VPMM_PowerSta_enum/1 -> [VPMM_PowerSta_enum]
  VPMM_PwrStaSW_enum/1 -> [VPMM_PwrStaSW_enum]
  [VINP_RR_AJAR_SW] -> Switch11/3
  Data Type Conversion9/1 -> Relational Operator8/2, Switch2/3
  Relational Operator8/1 -> Switch2/2
  Data Type Conversion2/1 -> Add3/2
  [VDDM_RRDoorSWHiLoCount_enum] -> Relational Operator1/1
  [VDDM_RRDoorSWHiLoCount_enum] -> Add2/1
  Data Type Conversion7/1 -> [VDDM_RRDoorSWfail_cnt]
  Relational Operator13/1 -> Switch3/2
  Data Type Conversion1/1 -> Relational Operator13/2, Switch3/3
  Data Type Conversion8/1 -> Switch9/1
  DTC_Info/1 -> VDDM_RRDoorSWDTC_raw32/1  "VDDM_RRDoorSWDTC_raw32"
  [VDDM_RRDoorSWPass_flg] -> DTC_Info/2
  [VDDM_RRDoorSWCFS_flg] -> DTC_Info/3
  [VDDM_RRDoorSWDet_flg] -> DTC_Info/1
  [task_time_s] -> Divide1/2
  [task_time_s] -> Divide20/2
  [task_time_s] -> Divide/2
  [task_time_s] -> Test Detection Criteria1/2
  [task_time_s] -> Divide16/2
  [task_time_s] -> Divide7/2
  [task_time_s] -> Divide11/2
  Constant5/1 -> Test Detection Criteria1/3
  [DTC_clear_request] -> DTC_Info/4
  [DTC_clear_request] -> Switch4/2
  Switch4/1 -> Test Detection Criteria1/1
  Constant9/1 -> Switch4/1
